simulink model "adaptive_sliding_mode_controller_feedback_lin_ned"  (R2020a)
settings: Solver=ode1  StartTime=0.0  StopTime=50  FixedStep=0.01  RelTol=1e-3
model workspace (MAT data in the model file):
  kd = 0
  kp = 0
libraries: simulink x5, sharedutil x1
settings Model: Creator=Sebas  LastModifiedBy=Sebas
settings SolverCC: ConcurrentTasks=on  ZeroCrossAlgorithm=Adaptive  AlgebraicLoopSolver=LineSearch
settings DebuggingCC: MaskedZcDiagnostic=none  IgnoredZcDiagnostic=none

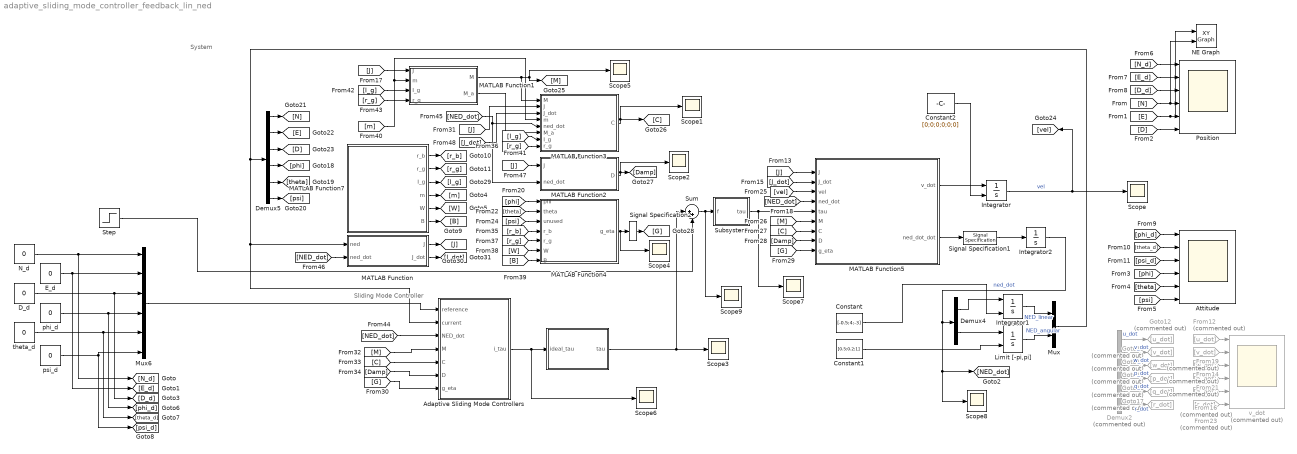
== system adaptive_sliding_mode_controller_feedback_lin_ned ==
  note: System
  note: Sliding Mode Controller
  " " : Subsystem
  Adaptive Sliding Mode Controllers : Subsystem  mask(6 DOF Adaptive Sliding Mode Controller){surge_k=0.3, sway_k=0.3, heave_k=0, roll_k=0, pitch_k=0, yaw_k=0, lambda_surge=2, lambda_sway=2, lambda_heave=1, lambda_roll=1, lambda_pitch=1, lambda_yaw=3, k_alpha_surge=0.5, k_alpha_sway=0.4, k_alpha_heave=0.1, k_alpha_roll=0.1, k_alpha_pitch=3, k_alpha_yaw=1.6, miu_surge=0.016, miu_sway=0.014, miu_heave=0.001, miu_roll=0.01, miu_pitch=0.01, miu_yaw=0.0036, Kmin_surge=0.01, Kmin_sway=0.01, Kmin_heave=0.05, Kmin_roll=0.01, Kmin_pitch=0.01, Kmin_yaw=0.01}
      mask prompts: surge_k "Surge"; sway_k "Sway"; heave_k "Heave"; roll_k "Roll"; pitch_k "Pitch"; yaw_k "Yaw"
      mask help: Implementation of 6 Adaptive Sliding Mode Controllers for each degree of freedom
      mask DialogControl Container5 Prompt: K2 Gains
      mask DialogControl Container13 Prompt: Adaptation Law for K1
      mask DialogControl Container11 Prompt: Adaptive rates
      mask DialogControl Container10 Prompt: Miu threshold
      mask DialogControl Container16 Prompt: Minimum gains
  Attitude : Scope  NumInputPorts=6
  Constant : Constant  Value=[-0.5;4;-3]
  Constant1 : Constant  Value=[0.5;0.2;1]
  Constant2 : Constant  Value=[0;0;0;0;0;0]
  D_d : Constant  Value=0
  Demux2 : Demux  Commented=on  Outputs=6
  Demux4 : Demux  Outputs=2
  Demux5 : Demux  Outputs=6
  E_d : Constant  Value=0
  From12 : From  Commented=on  GotoTag=u_dot
  From14 : From  Commented=on  GotoTag=w_dot
  From16 : From  Commented=on  GotoTag=q_dot
  From19 : From  Commented=on  GotoTag=v_dot
  From21 : From  Commented=on  GotoTag=p_dot
  From23 : From  Commented=on  GotoTag=r_dot
  Goto12 : Goto  Commented=on  GotoTag=u_dot
  Goto13 : Goto  Commented=on  GotoTag=v_dot
  Goto14 : Goto  Commented=on  GotoTag=w_dot
  Goto15 : Goto  Commented=on  GotoTag=p_dot
  Goto16 : Goto  Commented=on  GotoTag=q_dot
  Goto17 : Goto  Commented=on  GotoTag=r_dot
  Integrator : Integrator  InitialConditionSource=external
  Integrator1 : Integrator  InitialConditionSource=external
  Integrator2 : Integrator
  Limit [-pi,pi] : Integrator  InitialConditionSource=external  WrapState=on
  MATLAB Function : MATLAB Function  TreatAsAtomicUnit=on
  MATLAB Function1 : MATLAB Function  TreatAsAtomicUnit=on
  MATLAB Function2 : MATLAB Function  TreatAsAtomicUnit=on
  MATLAB Function3 : MATLAB Function  TreatAsAtomicUnit=on
  MATLAB Function4 : MATLAB Function  TreatAsAtomicUnit=on
  MATLAB Function5 : MATLAB Function  TreatAsAtomicUnit=on
  MATLAB Function7 : MATLAB Function  TreatAsAtomicUnit=on
  Mux : Mux  Inputs=2
  Mux6 : Mux  Inputs=6
  NE Graph : simulink/Sinks/XY Graph  xmin=-1  xmax=5  ymin=-1  ymax=2  st=-1
  N_d : Constant  Value=0
  Position : Scope  NumInputPorts=6
  Scope{,1..9} (10 alike) : Scope
  Signal Specification1 : SignalSpecification  Dimensions=6
  Signal Specification2 : SignalSpecification  Dimensions=6
  Step : Step  Time=20  After=[50;50;50;5;5;5]  SampleTime=0
  Subsystem : Subsystem
  Sum : Sum  Inputs=|++
  phi_d : Constant  Value=0
  psi_d : Constant  Value=0
  theta_d : Constant  Value=0
  v_dot : Scope  Commented=on  NumInputPorts=6
  wires:
  [N_d] -> Position/1
  [E_d] -> Position/2
  [D_d] -> Position/3
  [N] -> Position/4, NE Graph/2
  [D] -> Position/6
  [E] -> Position/5, NE Graph/1
  [phi_d] -> Attitude/1
  [phi] -> Attitude/4
  [psi_d] -> Attitude/3
  [theta] -> Attitude/5
  [psi] -> Attitude/6
  [theta_d] -> Attitude/2
  From12/1 -> v_dot/1
  From19/1 -> v_dot/2
  From14/1 -> v_dot/3
  From21/1 -> v_dot/4
  From16/1 -> v_dot/5
  From23/1 -> v_dot/6
  Demux2/1 -> Goto12/1  "u_dot"
  Demux2/5 -> Goto16/1  "q_dot"
  Demux2/3 -> Goto14/1  "w_dot"
  Demux2/6 -> Goto17/1  "r_dot"
  Demux2/4 -> Goto15/1  "p_dot"
  Demux2/2 -> Goto13/1  "v_dot"
  D_d/1 -> Mux6/3, [D_d]
  theta_d/1 -> Mux6/5, [theta_d]
  phi_d/1 -> Mux6/4, [phi_d]
  E_d/1 -> Mux6/2, [E_d]
  N_d/1 -> Mux6/1, [N_d]
  psi_d/1 -> [psi_d], Mux6/6
  Integrator/1 -> Scope/1, [vel]  "vel"
  Mux6/1 -> Adaptive Sliding Mode Controllers/1("reference ")
  Adaptive Sliding Mode Controllers/1(i_tau) -> Scope6/1, " "/1(ideal_tau)
  Step/1 -> Sum/2
  Sum/1 -> Scope9/1, Subsystem/1(f)
  MATLAB Function1/2(M_a) -> MATLAB Function3/6(M_a)
  Subsystem/1(tau) -> Scope7/1, MATLAB Function5/5(tau)
  Demux5/4 -> [phi]
  Demux5/5 -> [theta]
  Demux5/6 -> [psi]
  Demux5/2 -> [E]
  Demux5/1 -> [N]
  Demux5/3 -> [D]
  [NED_dot] -> MATLAB Function2/2(ned_dot), MATLAB Function3/5(ned_dot)
  [phi] -> MATLAB Function4/1(phi)
  [theta] -> MATLAB Function4/2(theta)
  [psi] -> MATLAB Function4/3(unused)
  [vel] -> MATLAB Function5/3(vel)
  MATLAB Function1/1(M) -> MATLAB Function3/1(M), [M], Scope5/1
  [M] -> MATLAB Function5/6(M)
  MATLAB Function3/1(C) -> Scope1/1, [C]
  [C] -> MATLAB Function5/7(C)
  MATLAB Function2/1(D) -> Scope2/1, [Damp]
  [Damp] -> MATLAB Function5/8(D)
  MATLAB Function4/1(g_eta) -> Signal Specification2/1, Scope4/1
  [G] -> MATLAB Function5/9(g_eta)
  [G] -> Adaptive Sliding Mode Controllers/7(g_eta)
  Mux/1 -> MATLAB Function/1(ned), Adaptive Sliding Mode Controllers/2(current), Demux5/1
  [C] -> Adaptive Sliding Mode Controllers/5(C)
  [Damp] -> Adaptive Sliding Mode Controllers/6(D)
  [M] -> Adaptive Sliding Mode Controllers/4(M)
  Constant2/1 -> Integrator/2
  MATLAB Function7/2(r_g) -> [r_g]
  MATLAB Function7/1(r_b) -> [r_b]
  MATLAB Function7/3(I_g) -> [I_g]
  MATLAB Function7/4(m) -> [m]
  MATLAB Function7/5(W) -> [W]
  MATLAB Function7/6(B) -> [B]
  [r_b] -> MATLAB Function4/4(r_b)
  [I_g] -> MATLAB Function3/7(I_g)
  [r_g] -> MATLAB Function4/5(r_g)
  [W] -> MATLAB Function4/6(W)
  [B] -> MATLAB Function4/7(B)
  [m] -> MATLAB Function3/4(m), MATLAB Function1/2(m)
  [r_g] -> MATLAB Function3/8(r_g)
  [I_g] -> MATLAB Function1/3(I_g)
  [r_g] -> MATLAB Function1/4(r_g)
  " "/1(tau) -> Scope3/1, Sum/1
  [NED_dot] -> Adaptive Sliding Mode Controllers/3(NED_dot)
  MATLAB Function5/1(v_dot) -> Integrator/1
  Constant1/1 -> Limit [-pi,pi]/2
  Constant/1 -> Integrator1/2
  Demux4/1 -> Integrator1/1
  Limit [-pi,pi]/1 -> Mux/2  "NED_angular"
  Integrator1/1 -> Mux/1  "NED_linear"
  Demux4/2 -> Limit [-pi,pi]/1
  Integrator2/1 -> [NED_dot], Scope8/1, Demux4/1  "ned_dot"
  [NED_dot] -> MATLAB Function5/4(ned_dot)
  MATLAB Function5/2(ned_dot_dot) -> Signal Specification1/1
  Signal Specification1/1 -> Integrator2/1
  Signal Specification2/1 -> [G]
  [NED_dot] -> MATLAB Function/2(ned_dot)
  MATLAB Function/1(J) -> [J]
  MATLAB Function/2(J_dot) -> [J_dot]
  [J] -> MATLAB Function5/1(J)
  [J_dot] -> MATLAB Function5/2(J_dot)
  [J] -> MATLAB Function1/1(J)
  [J] -> MATLAB Function2/1(J)
  [J] -> MATLAB Function3/2(J)
  [J_dot] -> MATLAB Function3/3(J_dot)

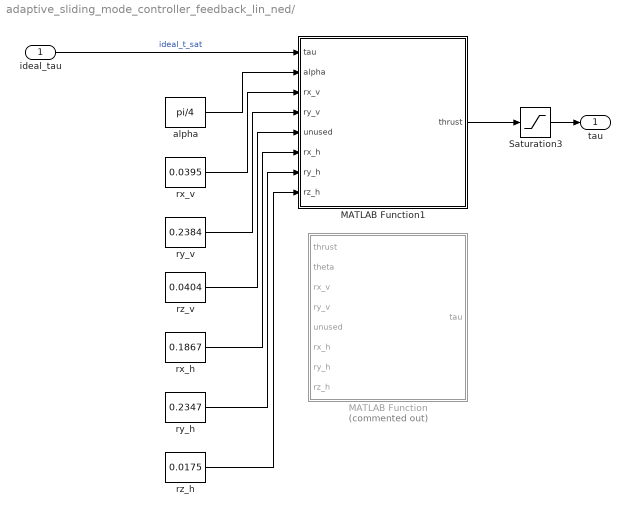
== system adaptive_sliding_mode_controller_feedback_lin_ned/  ==
  ideal_tau : Inport
  MATLAB Function : MATLAB Function  Commented=on  TreatAsAtomicUnit=on
  MATLAB Function1 : MATLAB Function  TreatAsAtomicUnit=on
  Saturation3 : Saturate  UpperLimit=35  LowerLimit=-35
  alpha : Constant  Value=pi/4
  rx_h : Constant  Value=0.1867
  rx_v : Constant  Value=0.0395
  ry_h : Constant  Value=0.2347
  ry_v : Constant  Value=0.2384
  rz_h : Constant  Value=0.0175
  rz_v : Constant  Value=0.0404
  tau : Outport
  wires:
  ideal_tau/1 -> MATLAB Function1/1(tau)  "ideal_t_sat"
  MATLAB Function1/1(thrust) -> Saturation3/1
  Saturation3/1 -> tau/1
  rx_v/1 -> MATLAB Function1/3(rx_v)
  alpha/1 -> MATLAB Function1/2(alpha)
  rx_h/1 -> MATLAB Function1/6(rx_h)
  ry_h/1 -> MATLAB Function1/7(ry_h)
  rz_h/1 -> MATLAB Function1/8(rz_h)
  ry_v/1 -> MATLAB Function1/4(ry_v)
  rz_v/1 -> MATLAB Function1/5(unused)

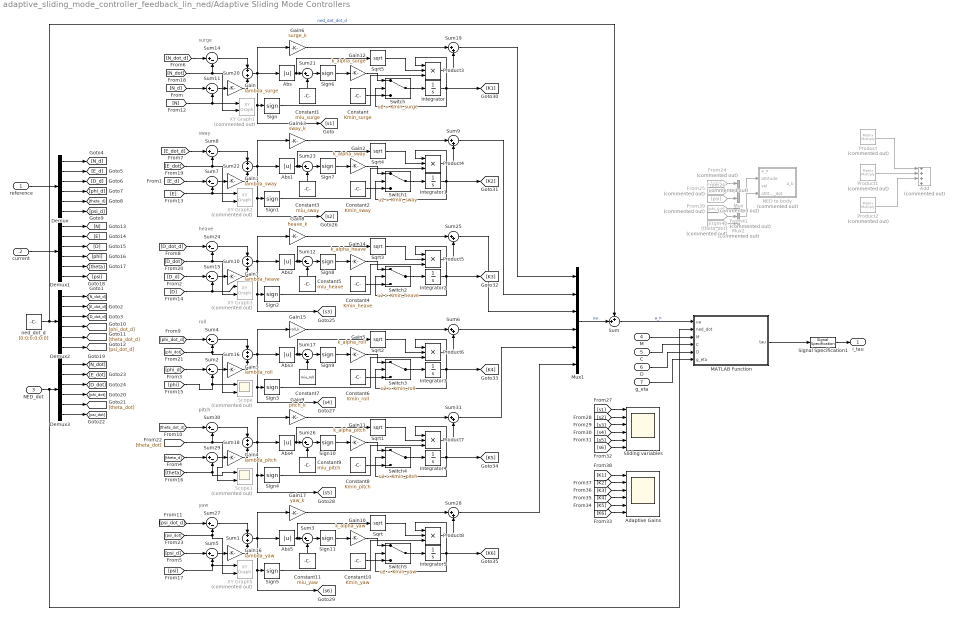
== system adaptive_sliding_mode_controller_feedback_lin_ned/Adaptive Sliding Mode Controllers ==
  note: surge
  note: sway
  note: heave
  note: roll
  note: pitch
  note: yaw
  "reference " : Inport
  current : Inport  Port=2
  NED_dot : Inport  Port=3
  M : Inport  Port=4
  C : Inport  Port=5
  D : Inport  Port=6
  g_eta : Inport  Port=7
  Abs{,1..5} (6 alike) : Abs
  Adaptive Gains : Scope  NumInputPorts=6
  Add : Sum  Commented=on  Inputs=4
  Constant : Constant  Value=Kmin_surge
  Constant1 : Constant  Value=miu_surge
  Constant10 : Constant  Value=Kmin_yaw
  Constant11 : Constant  Value=miu_yaw
  Constant2 : Constant  Value=Kmin_sway
  Constant3 : Constant  Value=miu_sway
  Constant4 : Constant  Value=Kmin_heave
  Constant5 : Constant  Value=miu_heave
  Constant6 : Constant  Value=Kmin_roll
  Constant7 : Constant  Value=miu_roll
  Constant8 : Constant  Value=Kmin_pitch
  Constant9 : Constant  Value=miu_pitch
  Demux{,1..3} (4 alike) : Demux  Outputs=6
  From24 : From  Commented=on  GotoTag=phi
  From25 : From  Commented=on  GotoTag=theta
  From26 : From  Commented=on  GotoTag=psi
  From39 : From  Commented=on  GotoTag=phi_dot
  From40 : From  Commented=on  GotoTag=theta_dot
  From41 : From  Commented=on  GotoTag=psi_dot
  Gain : Gain  Gain=lambda_surge
  Gain1 : Gain  Gain=lambda_sway
  Gain10 : Gain  Gain=k_alpha_yaw
  Gain11 : Gain  Gain=k_alpha_pitch
  Gain12 : Gain  Gain=k_alpha_surge
  Gain13 : Gain  Gain=sway_k
  Gain14 : Gain  Gain=k_alpha_heave
  Gain15 : Gain  Gain=roll_k
  Gain16 : Gain  Gain=lambda_yaw
  Gain17 : Gain  Gain=yaw_k
  Gain2 : Gain  Gain=k_alpha_sway
  Gain3 : Gain  Gain=lambda_roll
  Gain4 : Gain  Gain=lambda_pitch
  Gain5 : Gain  Gain=k_alpha_roll
  Gain6 : Gain  Gain=surge_k
  Gain7 : Gain  Gain=lambda_heave
  Gain8 : Gain  Gain=heave_k
  Gain9 : Gain  Gain=pitch_k
  Integrator{,1..5} (6 alike) : Integrator
  MATLAB Function : MATLAB Function  TreatAsAtomicUnit=on
  Mux : Mux  Commented=on  Inputs=3
  Mux1 : Mux  Inputs=6
  Mux2 : Mux  Commented=on  Inputs=3
  NED to body : Subsystem  Commented=on
  Product : Product  Commented=on  Multiplication=Matrix(*)
  Product1 : Product  Commented=on  Multiplication=Matrix(*)
  Product2 : Product  Commented=on  Multiplication=Matrix(*)
  Product{3..8} (6 alike) : Product  Inputs=3
  Scope : Scope  Commented=on  NumInputPorts=2
  Scope1 : Scope  Commented=on  NumInputPorts=2
  Sign{,1..11} (12 alike) : Signum  ZeroCross=off
  Signal Specification1 : SignalSpecification  Dimensions=6
  Sliding variables : Scope  NumInputPorts=6
  Sqrt{,1..5} (6 alike) : Sqrt  SaturateOnIntegerOverflow=on
  Sum : Sum  Inputs=++|
  Sum{1,10,16,18,20,22} (6 alike) : Sum
  Sum{2..5,7..8,11..12,14..15,17,21,23..24,26..27,29..30} (18 alike) : Sum  Inputs=|+-
  Sum{6,9,19,25,28,31} (6 alike) : Sum  Inputs=|++
  Switch : Switch  Criteria=u2 > Threshold  Threshold=Kmin_surge
  Switch1 : Switch  Criteria=u2 > Threshold  Threshold=Kmin_sway
  Switch2 : Switch  Criteria=u2 > Threshold  Threshold=Kmin_heave
  Switch3 : Switch  Criteria=u2 > Threshold  Threshold=Kmin_roll
  Switch4 : Switch  Criteria=u2 > Threshold  Threshold=Kmin_pitch
  Switch5 : Switch  Criteria=u2 > Threshold  Threshold=Kmin_yaw
  XY Graph1 : simulink/Sinks/XY Graph  Commented=on  xmin=-1  xmax=5  ymin=-1  ymax=1  st=-1
  XY Graph2 : simulink/Sinks/XY Graph  Commented=on  xmin=-1  xmax=5  ymin=-2  ymax=0.5  st=-1
  XY Graph3 : simulink/Sinks/XY Graph  Commented=on  xmin=-1  xmax=1  ymin=-1  ymax=1  st=-1
  XY Graph5 : simulink/Sinks/XY Graph  Commented=on  xmin=-1  xmax=1  ymin=-1  ymax=1  st=-1
  ned_dot_d : Constant  Value=[0;0;0;0;0;0]
  i_tau : Outport
  wires:
  current/1 -> Demux1/1
  Demux1/1 -> [N]
  "reference "/1 -> Demux/1
  Demux/1 -> [N_d]
  Demux1/2 -> [E]
  Demux/3 -> [D_d]
  Demux1/3 -> [D]
  Demux/4 -> [phi_d]
  Demux1/4 -> [phi]
  Demux/5 -> [theta_d]
  Demux1/5 -> [theta]
  Demux/6 -> [psi_d]
  Demux1/6 -> [psi]
  Demux2/1 -> [N_dot_d]
  Demux3/1 -> [N_dot]
  Demux2/2 -> [E_dot_d]
  Demux3/2 -> [E_dot]
  Demux2/3 -> [D_dot_d]
  Demux3/3 -> [D_dot]
  Demux2/4 -> [phi_dot_d]
  Demux3/4 -> [phi_dot]
  Demux2/5 -> [theta_dot_d]
  Demux3/5 -> [theta_dot]
  Demux3/6 -> [psi_dot]
  Demux2/6 -> [psi_dot_d]
  Demux/2 -> [E_d]
  ned_dot_d/1 -> Sum/1, Demux2/1  "ned_dot_dot_d"
  Mux1/1 -> Sum/2  "ua"
  M/1 -> MATLAB Function/3(M)
  C/1 -> MATLAB Function/4(C)
  D/1 -> MATLAB Function/5(D)
  g_eta/1 -> MATLAB Function/6(g_eta)
  NED_dot/1 -> MATLAB Function/2(ned_dot), Demux3/1
  [N] -> XY Graph1/1, Sum11/2
  Gain14/1 -> Switch2/1
  Gain15/1 -> Sum6/1
  Sign3/1 -> Product6/3
  Constant7/1 -> Sum17/2
  Sum20/1 -> [s1], Sign/1, Gain6/1, Abs/1
  Switch2/1 -> Integrator2/1
  Switch5/1 -> Integrator5/1
  Integrator4/1 -> [K5], Product7/1, Switch4/2
  Product6/1 -> Sum6/2
  [D_d] -> Sum15/1
  Gain3/1 -> Sum16/2
  Sign6/1 -> Gain12/1
  Sum16/1 -> [s4], Sign3/1, Gain15/1, Abs3/1
  Sum17/1 -> Sign9/1
  [phi] -> Sum2/2, Scope/1
  Sum26/1 -> Sign10/1
  Sum27/1 -> Sum1/1
  Abs3/1 -> Sqrt2/1, Sum17/1
  Constant3/1 -> Sum23/2
  [phi_dot] -> Scope/2, Sum4/2
  Gain5/1 -> Switch3/1
  Switch3/1 -> Integrator3/1
  Sign2/1 -> Product5/3
  Constant6/1 -> Switch3/3
  Gain1/1 -> Sum22/2
  Gain4/1 -> Sum18/2
  Sign4/1 -> Product7/3
  Constant9/1 -> Sum26/2
  Switch4/1 -> Integrator4/1
  Sum30/1 -> Sum18/1
  Gain12/1 -> Switch/1
  Gain8/1 -> Sum25/1
  Sign11/1 -> Gain10/1
  Gain/1 -> Sum20/2
  [N_d] -> Sum11/1
  Gain9/1 -> Sum31/1
  Integrator5/1 -> [K6], Product8/1, Switch5/2
  Gain16/1 -> Sum1/2
  Constant10/1 -> Switch5/3
  Switch1/1 -> Integrator1/1
  Sign5/1 -> Product8/3
  Sum1/1 -> Gain17/1, [s6], Sign5/1, Abs5/1
  Sum5/1 -> Gain16/1
  Integrator1/1 -> [K2], Switch1/2, Product4/1
  Gain17/1 -> Sum28/1
  Abs2/1 -> Sqrt3/1, Sum12/1
  Sum8/1 -> Sum22/1
  [psi] -> XY Graph5/1, Sum5/2
  Constant11/1 -> Sum3/2
  Sum4/1 -> Sum16/1
  Product8/1 -> Sum28/2
  Gain10/1 -> Switch5/1
  Constant/1 -> Switch/3
  Sum3/1 -> Sign11/1
  [psi_dot] -> XY Graph5/2, Sum27/2
  [theta] -> Scope1/1, Sum29/2
  Sign8/1 -> Gain14/1
  Sum12/1 -> Sign8/1
  Integrator2/1 -> [K3], Product5/1, Switch2/2
  [D] -> Sum15/2, XY Graph3/1
  Product5/1 -> Sum25/2
  Constant4/1 -> Switch2/3
  [theta_d] -> Sum29/1
  Gain7/1 -> Sum10/2
  Sum24/1 -> Sum10/1
  Sign1/1 -> Product4/3
  Abs1/1 -> Sqrt4/1, Sum23/1
  Sum22/1 -> Gain13/1, Abs1/1, [s2], Sign1/1
  Product3/1 -> Sum19/2
  Abs/1 -> Sqrt5/1, Sum21/1
  [psi_dot_d] -> Sum27/1
  Product4/1 -> Sum9/2
  Integrator/1 -> [K1], Switch/2, Product3/1
  Sum19/1 -> Mux1/1
  [theta_dot_d] -> Sum30/1
  [phi_dot_d] -> Sum4/1
  Sum14/1 -> Sum20/1
  [N_dot] -> Sum14/2, XY Graph1/2
  Constant2/1 -> Switch1/3
  Sum6/1 -> Mux1/4
  Product7/1 -> Sum31/2
  Sum25/1 -> Mux1/3
  Gain13/1 -> Sum9/1
  Gain2/1 -> Switch1/1
  Sum21/1 -> Sign6/1
  Gain11/1 -> Switch4/1
  Sum15/1 -> Gain7/1
  Sum7/1 -> Gain1/1
  [E] -> XY Graph2/1, Sum7/2
  Sum9/1 -> Mux1/2
  [psi_d] -> Sum5/1
  Sign10/1 -> Gain11/1
  Gain6/1 -> Sum19/1
  [N_dot_d] -> Sum14/1
  Sum28/1 -> Mux1/6
  [E_dot] -> XY Graph2/2, Sum8/2
  Switch/1 -> Integrator/1
  Sum11/1 -> Gain/1
  Integrator3/1 -> [K4], Product6/1, Switch3/2
  Sign9/1 -> Gain5/1
  Sum18/1 -> [s5], Sign4/1, Gain9/1, Abs4/1
  [phi_d] -> Sum2/1
  [E_dot_d] -> Sum8/1
  Constant8/1 -> Switch4/3
  Sum23/1 -> Sign7/1
  Sum31/1 -> Mux1/5
  Abs5/1 -> Sqrt/1, Sum3/1
  Sum29/1 -> Gain4/1
  [theta_dot] -> Scope1/2, Sum30/2
  Sum10/1 -> [s3], Sign2/1, Gain8/1, Abs2/1
  [E_d] -> Sum7/1
  Constant1/1 -> Sum21/2
  Sign7/1 -> Gain2/1
  Constant5/1 -> Sum12/2
  Sign/1 -> Product3/3
  [D_dot_d] -> Sum24/1
  Abs4/1 -> Sqrt1/1, Sum26/1
  [D_dot] -> Sum24/2, XY Graph3/2
  [s1] -> Sliding variables/1
  [s2] -> Sliding variables/2
  [s3] -> Sliding variables/3
  [s4] -> Sliding variables/4
  [s5] -> Sliding variables/5
  [s6] -> Sliding variables/6
  [K6] -> Adaptive Gains/6
  [K5] -> Adaptive Gains/5
  [K4] -> Adaptive Gains/4
  [K3] -> Adaptive Gains/3
  [K2] -> Adaptive Gains/2
  [K1] -> Adaptive Gains/1
  Sqrt5/1 -> Product3/2
  Sqrt4/1 -> Product4/2
  Sqrt3/1 -> Product5/2
  Sqrt2/1 -> Product6/2
  Sqrt1/1 -> Product7/2
  Sqrt/1 -> Product8/2
  MATLAB Function/1(tau) -> Signal Specification1/1
  Signal Specification1/1 -> i_tau/1
  Sum2/1 -> Gain3/1
  From26/1 -> Mux/3
  Mux2/1 -> NED to body/4(attitude_dot)
  From40/1 -> Mux2/2
  From25/1 -> Mux/2
  Mux/1 -> NED to body/2(attitude)
  From39/1 -> Mux2/1
  From24/1 -> Mux/1
  From41/1 -> Mux2/3
  Product1/1 -> Add/2
  Product/1 -> Add/1
  Product2/1 -> Add/3
  Sum/1 -> MATLAB Function/1(ua)  "a_n"

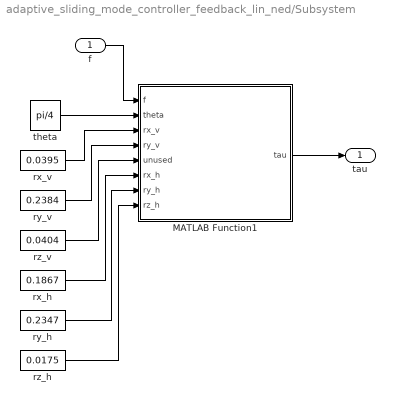
== system adaptive_sliding_mode_controller_feedback_lin_ned/Subsystem ==
  f : Inport
  MATLAB Function1 : MATLAB Function  TreatAsAtomicUnit=on
  rx_h : Constant  Value=0.1867
  rx_v : Constant  Value=0.0395
  ry_h : Constant  Value=0.2347
  ry_v : Constant  Value=0.2384
  rz_h : Constant  Value=0.0175
  rz_v : Constant  Value=0.0404
  theta : Constant  Value=pi/4
  tau : Outport
  wires:
  rz_v/1 -> MATLAB Function1/5(unused)
  ry_h/1 -> MATLAB Function1/7(ry_h)
  f/1 -> MATLAB Function1/1(f)
  MATLAB Function1/1(tau) -> tau/1
  rx_h/1 -> MATLAB Function1/6(rx_h)
  theta/1 -> MATLAB Function1/2(theta)
  rx_v/1 -> MATLAB Function1/3(rx_v)
  rz_h/1 -> MATLAB Function1/8(rz_h)
  ry_v/1 -> MATLAB Function1/4(ry_v)

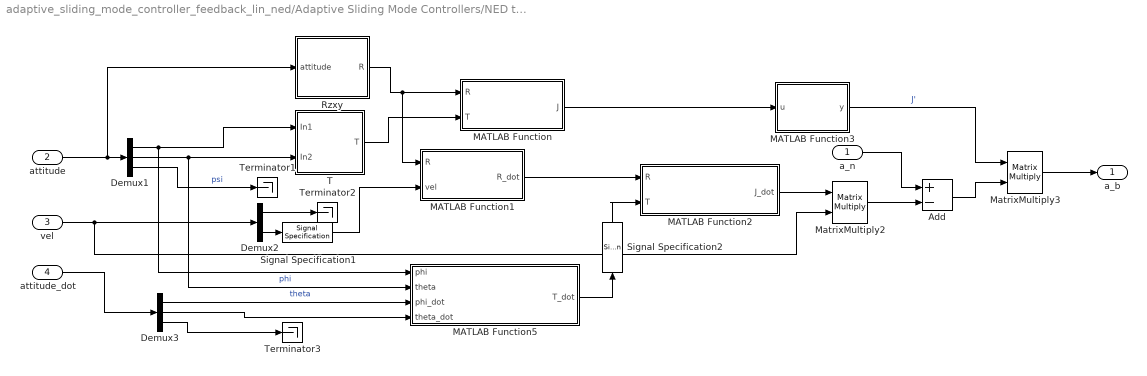
== system adaptive_sliding_mode_controller_feedback_lin_ned/Adaptive Sliding Mode Controllers/NED to body ==
  a_n : Inport
  attitude : Inport  Port=2
  vel : Inport  Port=3
  attitude_dot : Inport  Port=4
  Add : Sum  Inputs=+-
  Demux1 : Demux  Outputs=3
  Demux2 : Demux  Outputs=2
  Demux3 : Demux  Outputs=3
  MATLAB Function : MATLAB Function  TreatAsAtomicUnit=on
  MATLAB Function1 : MATLAB Function  TreatAsAtomicUnit=on
  MATLAB Function2 : MATLAB Function  TreatAsAtomicUnit=on
  MATLAB Function3 : MATLAB Function  TreatAsAtomicUnit=on
  MATLAB Function5 : MATLAB Function  TreatAsAtomicUnit=on
  MatrixMultiply2 : Product  Multiplication=Matrix(*)
  MatrixMultiply3 : Product  Multiplication=Matrix(*)
  Rzxy : Subsystem
  Signal Specification1 : SignalSpecification  Dimensions=3
  Signal Specification2 : SignalSpecification  Dimensions=[3,3]
  T : Subsystem
  Terminator1 : Terminator
  Terminator2 : Terminator
  Terminator3 : Terminator
  a_b : Outport
  wires:
  a_n/1 -> Add/1
  attitude/1 -> Demux1/1, Rzxy/1(attitude)
  Demux1/1 -> T/1(In1), MATLAB Function5/1(phi)  "phi"
  Demux1/2 -> T/2(In2), MATLAB Function5/2(theta)  "theta"
  MATLAB Function/1(J) -> MATLAB Function3/1(u)
  Demux1/3 -> Terminator1/1  "psi"
  Rzxy/1(R) -> MATLAB Function1/1(R), MATLAB Function/1(R)
  T/1(T) -> MATLAB Function/2(T)
  MATLAB Function1/1(R_dot) -> MATLAB Function2/1(R)
  Demux2/1 -> Terminator2/1
  MatrixMultiply2/1 -> Add/2
  Add/1 -> MatrixMultiply3/2
  MatrixMultiply3/1 -> a_b/1
  Demux2/2 -> Signal Specification1/1
  MATLAB Function3/1(y) -> MatrixMultiply3/1  "J'"
  vel/1 -> Demux2/1, MatrixMultiply2/2
  Signal Specification1/1 -> MATLAB Function1/2(vel)
  MATLAB Function2/1(J_dot) -> MatrixMultiply2/1
  MATLAB Function5/1(T_dot) -> Signal Specification2/1
  attitude_dot/1 -> Demux3/1
  Demux3/3 -> Terminator3/1
  Demux3/1 -> MATLAB Function5/3(phi_dot)
  Demux3/2 -> MATLAB Function5/4(theta_dot)
  Signal Specification2/1 -> MATLAB Function2/2(T)

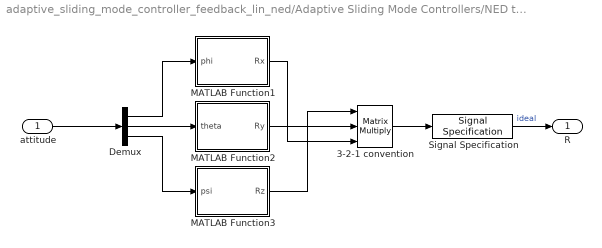
== system adaptive_sliding_mode_controller_feedback_lin_ned/Adaptive Sliding Mode Controllers/NED to body/Rzxy ==
  attitude : Inport
  3-2-1 convention : Product  Inputs=3  Multiplication=Matrix(*)
  Demux : Demux  Outputs=3
  MATLAB Function1 : MATLAB Function  TreatAsAtomicUnit=on
  MATLAB Function2 : MATLAB Function  TreatAsAtomicUnit=on
  MATLAB Function3 : MATLAB Function  TreatAsAtomicUnit=on
  Signal Specification : SignalSpecification  Dimensions=[3,3]
  R : Outport
  wires:
  Demux/1 -> MATLAB Function1/1(phi)
  MATLAB Function3/1(Rz) -> 3-2-1 convention/1
  MATLAB Function2/1(Ry) -> 3-2-1 convention/2
  Demux/3 -> MATLAB Function3/1(psi)
  MATLAB Function1/1(Rx) -> 3-2-1 convention/3
  3-2-1 convention/1 -> Signal Specification/1
  attitude/1 -> Demux/1
  Demux/2 -> MATLAB Function2/1(theta)
  Signal Specification/1 -> R/1  "ideal"

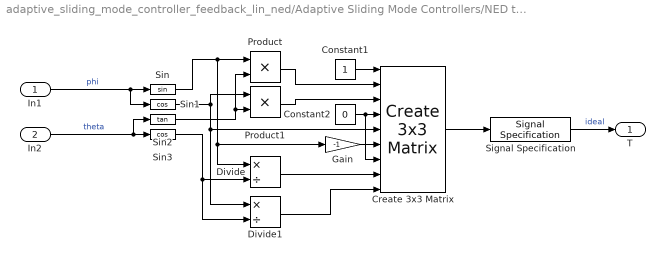
== system adaptive_sliding_mode_controller_feedback_lin_ned/Adaptive Sliding Mode Controllers/NED to body/T ==
  In1 : Inport
  In2 : Inport  Port=2
  Constant1 : Constant
  Constant2 : Constant  Value=0
  Create 3x3 Matrix : sharedutil/Create 3x3 Matrix  aMode=aMode
      settings: SourceProductBaseCode=AE,PW,MT,VE,VP
  Divide : Product  Inputs=*/
  Divide1 : Product  Inputs=*/
  Gain : Gain  Gain=-1
  Product : Product
  Product1 : Product
  Signal Specification : SignalSpecification  Dimensions=[3,3]
  Sin : Trigonometry
  Sin1 : Trigonometry  Operator=cos
  Sin2 : Trigonometry  Operator=tan
  Sin3 : Trigonometry  Operator=cos
  T : Outport
  wires:
  Constant2/1 -> Create 3x3 Matrix/7, Create 3x3 Matrix/4
  Gain/1 -> Create 3x3 Matrix/6
  Divide1/1 -> Create 3x3 Matrix/9
  Product/1 -> Create 3x3 Matrix/2
  Sin1/1 -> Divide1/1, Create 3x3 Matrix/5, Product1/1
  In1/1 -> Sin1/1, Sin/1  "phi"
  Sin2/1 -> Product/2, Product1/2
  Divide/1 -> Create 3x3 Matrix/8
  Product1/1 -> Create 3x3 Matrix/3
  Sin3/1 -> Divide1/2, Divide/2
  In2/1 -> Sin2/1, Sin3/1  "theta"
  Sin/1 -> Gain/1, Divide/1, Product/1
  Constant1/1 -> Create 3x3 Matrix/1
  Create 3x3 Matrix/1 -> Signal Specification/1
  Signal Specification/1 -> T/1  "ideal"

== matlab function adaptive_sliding_mode_controller_feedback_lin_ned/Adaptive Sliding Mode Controllers/NED to body/MATLAB Function2 ==
  data: R input; J_dot output; T input
function J_dot = diff_transform_matrix(R,T)
J_dot = [R          zeros(3);
         zeros(3)    T];

== matlab function adaptive_sliding_mode_controller_feedback_lin_ned/Adaptive Sliding Mode Controllers/NED to body/MATLAB Function3 ==
  data: u input; y output
function y = fcn(u)
y = inv(u);

== matlab function adaptive_sliding_mode_controller_feedback_lin_ned/ /MATLAB Function1 ==
  data: tau input; thrust output; alpha input; rx_v input; ry_v input; unused input; rx_h input; ry_h input; rz_h input
function thrust = thrust_allocation(tau, alpha, rx_v, ry_v, ~, rx_h, ry_h, rz_h)
% Mapping matrix
T = [cos(alpha) cos(alpha) -cos(alpha) -cos(alpha) 0 0;
     -sin(alpha) sin(alpha) -sin(alpha) sin(alpha) 0 0;
     0 0 0 0 -1 -1;
     -sin(alpha)*rz_h sin(alpha)*rz_h -sin(alpha)*rz_h sin(alpha)*rz_h -ry_v ry_v;
     -cos(alpha)*rz_h -cos(alpha)*rz_h cos(alpha)*rz_h cos(alpha)*rz_h -rx_v rx_v;
     -(rx_h*sin(alpha)+ry_h*cos(alpha)) (rx_h*sin(alpha)+ry_h*cos(alpha)) (rx_h*sin(alpha)+ry_h*cos(alpha)) -(rx_h*sin(alpha)+ry_h*cos(alpha)) 0 0
    ];
% Control input with Moore–Penrose pseudo-inverse
t = pinv(T)*tau;
thrust = t;

== matlab function adaptive_sliding_mode_controller_feedback_lin_ned/MATLAB Function2 ==
  data: J input; ned_dot input; D output
function D = Damping(J,ned_dot)
% Linear damping coefficients
X_u = -0.3431;
Y_v = 0.0518;
Z_w = -0.5841;
K_p = 0.0064;
M_q = 0.04;
N_r = -0.1063;

% Cuadratic damping coefficients
X_uu = -111.7397;
Y_vv = -44.4058;
Z_ww = -157.1951;
K_pp = -0.4634;
M_qq = -0.2902;
N_rr = -2.2897;

% Linear damping matrix
D_lin = -diag([X_u Y_v Z_w K_p M_q N_r]);

% Cuadratic Damping matrix
D_cuad = -diag([X_uu*abs(ned_dot(1)) Y_vv*abs(ned_dot(2)) Z_ww*abs(ned_dot(3)) ...
               K_pp*abs(ned_dot(4)) M_qq*abs(ned_dot(5)) N_rr*abs(ned_dot(6))]);

%Damping matrix
D = D_lin + D_cuad;

D = D/J;

== matlab function adaptive_sliding_mode_controller_feedback_lin_ned/MATLAB Function3 ==
  data: M input; J input; J_dot input; m input; ned_dot input; C output; M_a input; I_g input; r_g input
function C = Coriolis(M, J, J_dot, m,ned_dot,M_a,I_g,r_g)
% Skew symmetric matrix
S = @(s) [0    -s(3) s(2);
          s(3) 0     -s(1);
          -s(2) s(1)  0    ];  

% Rigid-body Coriolis-centripetal Matrix
C_rb = [ zeros(3)             -m*S(ned_dot(1:3))-m*S(ned_dot(4:6))*S(r_g);
        -m*S(ned_dot(1:3))+m*S(r_g)*S(ned_dot(4:6))            -S(I_g*ned_dot(4:6))];

% Coreolis added mass matrix 
C_a = [ 0 0 0   0 -M_a(3,3)*ned_dot(3) M_a(2,2)*ned_dot(2) ;
        0 0 0   M_a(3,3)*ned_dot(3) 0 -M_a(1,1)*ned_dot(1) ;
        0 0 0  -M_a(2,2)*ned_dot(2) M_a(1,1)*ned_dot(1) 0  ;
        0 -M_a(3,3)*ned_dot(3) M_a(2,2)*ned_dot(2)  0 -M_a(6,6)*ned_dot(6) M_a(5,5)*ned_dot(5) ;
        M_a(3,3)*ned_dot(3) 0 -M_a(1,1)*ned_dot(1)  M_a(6,6)*ned_dot(6) 0 -M_a(4,4)*ned_dot(4) ;
       -M_a(2,2)*ned_dot(2) M_a(1,1)*ned_dot(1) 0   -M_a(5,5)*ned_dot(5) M_a(4,4)*ned_dot(4) 0  ];

% Coreolis matrix
C = C_rb + C_a;

C = -M*inv(J)*J_dot*inv(J) + C*inv(J);

== matlab function adaptive_sliding_mode_controller_feedback_lin_ned/MATLAB Function4 ==
  data: phi input; g_eta output; theta input; unused input; r_b input; r_g input; W input; B input
function g_eta = Restore(phi,theta,~,r_b,r_g,W,B)
% Restoring forces
g_eta = [ (W-B)*sin(theta);
          -(W-B)*cos(theta)*sin(phi);
          -(W-B)*cos(theta)*cos(phi);
          -(r_g(2)*W-r_b(2)*B)*cos(theta)*cos(phi) + (r_g(3)*W-r_b(3)*B)*cos(theta)*sin(phi);
           (r_g(3)*W-r_b(3)*B)*sin(theta)             + (r_g(1)*W-r_b(1)*B)*cos(theta)*cos(phi)
          -(r_g(1)*W-r_b(1)*B)*cos(theta)*sin(phi) - (r_g(2)*W-r_b(2)*B)*sin(theta)          ];

== matlab function adaptive_sliding_mode_controller_feedback_lin_ned/MATLAB Function5 ==
  data: v_dot output; J input; J_dot input; vel input; ned_dot input; tau input; M input; C input; D input; ned_dot_dot output; g_eta input
function [v_dot,ned_dot_dot] = Forward_dynamics(J, J_dot,vel,ned_dot,tau,M,C,D,g_eta) 
% viejo:
%f = J_dot*inv(J)*ned_dot - J*inv(M)*C*inv(J)*ned_dot - J*inv(M)*D*inv(J)*ned_dot - J*inv(M)*g_eta;
%g = J*inv(M);
 
f = -inv(M)*C*ned_dot - inv(M)*D*ned_dot - inv(M)*g_eta;
g = inv(M);

ned_dot_dot = f + g*tau;
v_dot = J\(ned_dot_dot - J_dot*inv(J)*ned_dot);

== matlab function adaptive_sliding_mode_controller_feedback_lin_ned/Adaptive Sliding Mode Controllers/MATLAB Function ==
  data: ua input; ned_dot input; tau output; M input; C input; D input; g_eta input
function tau  = control(ua,ned_dot,M,C,D,g_eta)
% viejo:
%f = J_dot*inv(J)*ned_dot - J*inv(M)*C*inv(J)*ned_dot - J*inv(M)*D*inv(J)*ned_dot - J*inv(M)*g_eta;
%g = J*inv(M);
 
f_neg = inv(M)*C*ned_dot - inv(M)*D*ned_dot - inv(M)*g_eta;

tau = M*(ua + f_neg);

== matlab function adaptive_sliding_mode_controller_feedback_lin_ned/MATLAB Function7 ==
  data: r_b output; r_g output; I_g output; m output; W output; B output
function [r_b,r_g,I_g,m,W,B] = System_parameters()
r_g = [0 0 0].';    % Distance from origin to center of mass
r_b = [0 0 -0.10726].';    % Distance from origin to center of buoyancy
I_g = [0.900121387  -0.000186482 0.0072251;
       -0.000186482 1.754494427  0.020319615;
       0.0072251    0.020319615  1.43389     ]; % Rigid-body inertia matrix
m = 24;
vol = 0.02306187;
W = m*9.81;
B = W*1.005; %1000*9.81*vol;

== matlab function adaptive_sliding_mode_controller_feedback_lin_ned/Adaptive Sliding Mode Controllers/NED to body/MATLAB Function5 ==
  data: phi input; T_dot output; theta input; phi_dot input; theta_dot input
function T_dot = Diff_trans_matrix(phi, theta, phi_dot, theta_dot)
T_dot = [ 0  sin(phi)*((sec(theta)^2))*theta_dot + cos(phi)*tan(theta)*phi_dot   cos(phi)*((sec(theta))^2)*theta_dot - sin(phi)*tan(theta)*phi_dot;
          0  -sin(phi)*phi_dot                                                   -cos(phi)*phi_dot;
          0  (cos(theta)*cos(phi)*phi_dot + sin(phi)*sin(theta)*theta_dot)/(cos(theta))^2    (-cos(theta)*sin(phi)*phi_dot + cos(phi)*sin(theta)*theta_dot)/(cos(theta))^2
        ];

== matlab function adaptive_sliding_mode_controller_feedback_lin_ned/MATLAB Function ==
  data: ned input; J output; J_dot output; ned_dot input
function [J, J_dot] = transforms(ned, ned_dot)
% Skew symmetric matrix
Skew = @(s) [0    -s(3) s(2);
          s(3) 0     -s(1);
          -s(2) s(1)  0    ];  
      
phi = ned(4);
theta = ned(5);
psi = ned(6);
      
% 3-2-1 rotation
R = [ cos(psi)*cos(theta) -sin(psi)*cos(phi) + cos(psi)*sin(theta)*sin(phi)   sin(psi)*sin(phi) + cos(psi)*cos(phi)*sin(theta);
      sin(psi)*cos(theta) cos(psi)*cos(phi) + sin(phi)*sin(theta)*sin(psi)    -cos(psi)*sin(phi) + sin(theta)*sin(psi)*cos(phi);
      -sin(theta) cos(theta)*sin(phi) cos(theta)*cos(phi) ];

T = [ 1 sin(phi)*tan(theta) cos(phi)*tan(theta);
      0 cos(phi)            -sin(phi)
      0 sin(phi)/cos(theta) cos(phi)/cos(theta) ];
  
J = [R          zeros(3);
     zeros(3)   T];

a = J\ned_dot;
R_dot = R*Skew(a);

phi_dot = ned_dot(4);
theta_dot = ned_dot(5);
%psi_dot = ned_dot(6);

T_dot = [ 0  sin(phi)*((sec(theta)^2))*theta_dot + cos(phi)*tan(theta)*phi_dot   cos(phi)*((sec(theta))^2)*theta_dot - sin(phi)*tan(theta)*phi_dot;
          0  -sin(phi)*phi_dot                                                   -cos(phi)*phi_dot;
          0  (cos(theta)*cos(phi)*phi_dot + sin(phi)*sin(theta)*theta_dot)/(cos(theta))^2    (-cos(theta)*sin(phi)*phi_dot + cos(phi)*sin(theta)*theta_dot)/(cos(theta))^2
        ];
    
J_dot = [R_dot         zeros(3);
         zeros(3)       T_dot];

== matlab function adaptive_sliding_mode_controller_feedback_lin_ned/Adaptive Sliding Mode Controllers/NED to body/Rzxy/MATLAB Function1 ==
  data: phi input; Rx output
function Rx = Rx(phi)
Rx = [ 1 0 0;
       0 cos(phi) -sin(phi);
       0 sin(phi) cos(phi); ];

== matlab function adaptive_sliding_mode_controller_feedback_lin_ned/MATLAB Function1 ==
  data: J input; m input; M output; M_a output; I_g input; r_g input
function [M,M_a] = Mass_Matrix(J,m,I_g,r_g)
% Skew symmetric matrix
S = @(s) [0    -s(3) s(2);
          s(3) 0     -s(1);
          -s(2) s(1)  0    ];  

% Rigid-Body Inertia Matrix
M_rb = [ m*eye(3)    -m*S(r_g);
         m*S(r_g)         I_g ];

% Added mass matrix
M_a = diag([16.8374 20.2748 35.3180 0.2165 0.6869 0.6157]);

% Mass matrix
M = M_rb + M_a;

M = M/J;

== matlab function adaptive_sliding_mode_controller_feedback_lin_ned/ /MATLAB Function ==
  data: thrust input; tau output; theta input; rx_v input; ry_v input; unused input; rx_h input; ry_h input; rz_h input
function tau = thrust_conversion(thrust, theta, rx_v, ry_v, ~, rx_h, ry_h, rz_h)
% Errores numericos. El input esta saturado a [100,-100], y estas salidas
% dan valores muchisimo mayores a 35 N c/u
tau = [0 0 0 0 0 0].';
% For surge
s_val = thrust(1)/cos(theta)/4;
tau(1) = tau(1)+s_val;
tau(2) = tau(2)+s_val;
tau(3) = tau(3)-s_val;
tau(4) = tau(4)-s_val;

% For sway
sw_val = thrust(2)/sin(theta)/4;
tau(1) = tau(1)-sw_val;
tau(2) = tau(2)+sw_val;
tau(3) = tau(3)-sw_val;
tau(4) = tau(4)+sw_val;

% For heave
tau(5) = tau(5)+(-thrust(3)/2);
tau(6) = tau(6)+(-thrust(3)/2);

% For yaw
y_val = thrust(6)/(rx_h*sin(theta)+ry_h*cos(theta))/4;
tau(1) = tau(1)-y_val;
tau(2) = tau(2)+y_val;
tau(3) = tau(3)+y_val;
tau(4) = tau(4)-y_val;

% K and M come as zero
% For K
if  thrust(4)~= 0
    %disp("K")
    k_val = (thrust(4)-(-tau(1)+tau(2)-tau(3)+tau(4))*sin(theta)*rz_h)/(2*ry_v);
    tau(5) = tau(5)-k_val;
    tau(6) = tau(6)+k_val;
end

% For M
if thrust(5) ~= 0
    %disp("M")
    M_val = (thrust(5)-(-tau(1)-tau(2)+tau(3)+tau(4))*cos(theta)*rz_h)/(2*rx_v);
    tau(5) = tau(5)-M_val;
    tau(6) = tau(6)+M_val;
end
disp(tau)

== matlab function adaptive_sliding_mode_controller_feedback_lin_ned/Adaptive Sliding Mode Controllers/NED to body/MATLAB Function ==
  data: R input; J output; T input
function J = transform_matrix(R,T)
J= [R          zeros(3);
     zeros(3)    T];

== matlab function adaptive_sliding_mode_controller_feedback_lin_ned/Subsystem/MATLAB Function1 ==
  data: tau output; f input; theta input; rx_v input; ry_v input; unused input; rx_h input; ry_h input; rz_h input
function tau = tau_conversion(f, theta, rx_v, ry_v, ~, rx_h, ry_h, rz_h)
tau = [0 0 0 0 0 0].';
tau(1) = (f(1)+f(2)-f(3)-f(4))*cos(theta);
tau(2) = (-f(1)+f(2)-f(3)+f(4))*sin(theta);
tau(3) = -(f(5)+f(6));
tau(4) = (f(6)-f(5))*ry_v + (-f(1)+f(2)-f(3)+f(4))*sin(theta)*rz_h;
tau(5) = (f(6)-f(5))*rx_v + (-f(1)-f(2)+f(3)+f(4))*cos(theta)*rz_h;
tau(6) = (-f(1)+f(2)+f(3)-f(4))*(rx_h*sin(theta)+ry_h*cos(theta));

== matlab function adaptive_sliding_mode_controller_feedback_lin_ned/Adaptive Sliding Mode Controllers/NED to body/Rzxy/MATLAB Function2 ==
  data: theta input; Ry output
function Ry = Ry(theta)
Ry = [ cos(theta) 0 sin(theta);
       0          1     0 ;
       -sin(theta) 0 cos(theta); ];

== matlab function adaptive_sliding_mode_controller_feedback_lin_ned/Adaptive Sliding Mode Controllers/NED to body/Rzxy/MATLAB Function3 ==
  data: psi input; Rz output
function Rz = Rz(psi)
Rz = [ cos(psi) -sin(psi) 0;
       sin(psi) cos(psi)  0;
       0        0         1];

== matlab function adaptive_sliding_mode_controller_feedback_lin_ned/Adaptive Sliding Mode Controllers/NED to body/MATLAB Function1 ==
  data: R input; vel input; R_dot output
function R_dot = Diff_Rot_matrix(R,vel)
% Skew symmetric matrix
a = [0    -vel(3) vel(2);
     vel(3) 0     -vel(1);
     -vel(2) vel(1)  0    ];
R_dot = R*a;
